simulink model "DAMPER"  (R2020a)
settings: Solver=VariableStepAuto  StartTime=0.0  StopTime=10  RelTol=1e-3
settings Model: Creator=naina  LastModifiedBy=naina

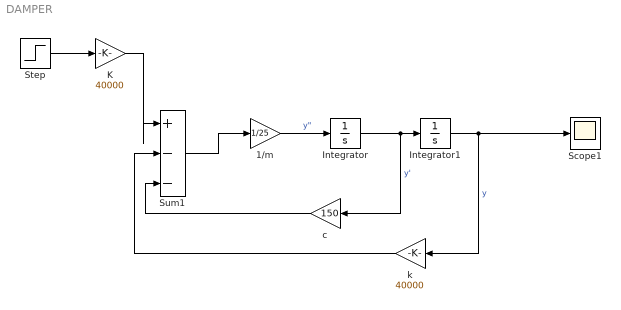
== system DAMPER ==
  1/m : Gain  Gain=1/25
  Integrator : Integrator
  Integrator1 : Integrator
  K : Gain  Gain=40000
  Scope1 : Scope
  Step : Step  SampleTime=0
  Sum1 : Sum  Inputs=|+--
  c : Gain  Gain=150
  k : Gain  Gain=40000
  wires:
  Integrator/1 -> c/1, Integrator1/1  "y'"
  Integrator1/1 -> k/1, Scope1/1  "y"
  1/m/1 -> Integrator/1  "y\""
  Sum1/1 -> 1/m/1
  Step/1 -> K/1
  K/1 -> Sum1/1
  c/1 -> Sum1/3
  k/1 -> Sum1/2
